simulink model "Mastership"  (R2013b)
settings: Solver=ode45  StartTime=0.0  StopTime=6e-4  RelTol=1e-3
(part 2 of 3)

== stateflow chart Mastership/MVBC/MVB3 ==
  state ClockManager [parallel]
    settings: executionOrder=1
    note: 描述：时钟管理模块，负责从主时钟（24Mhz）分频产生不同的时钟信号。同时负责过程数据
        | 更新时间戳的生成。
        | 通信方法：0.时钟频率24MHz, RST信号异步复位
        | 			1.3Mhz时钟输出：CLK_3Mhz
        | 			2.1Khz时钟输出：CLK_1Khz
        | 			3.时间戳输出：timeStamp（每1ms计数1次）
        | 假定情况：未考虑时钟同步提取问题，后期工作应加入设备间时钟同步模块
        | 作者：周彦钊
        | 最后修改者：周彦钊
        | 更新日期：2014.1.21
    state FreqDivider [parallel]
      settings: executionOrder=1
      note: 描述：分频器
      state Wait
        ClockManager.FreqDivider.Wait -> ClockManager.FreqDivider.Wait [order 1] : [!RST]
            | {Reset();}
      state Event
        (default) -> (junction 30)
        (junction 30) -> (junction 24) [order 1] : [counter_3M==4]
            | {CLK_3MHz=~CLK_3MHz
            | counter_3M=0;}
        (junction 30) -> (junction 33) [order 2]
        (junction 24) -> (junction 33)
        (junction 33) -> (junction 37) [order 1] : [counter_1K==12000]
            | {CLK_1KHz=~CLK_1KHz;
            | counter_1K=0;}
        (junction 33) -> (junction 386) [order 2]
        (junction 37) -> (junction 386)
        (junction 386) -> (junction 388) : [counter_BasicPeriod==100]
            | {basicPeriodStart = ~basicPeriodStart
            | counter_BasicPeriod = 0;}
      (default) -> ClockManager.FreqDivider.Wait : {Reset();}
      ClockManager.FreqDivider.Event -> ClockManager.FreqDivider.Wait
      ClockManager.FreqDivider.Wait -> ClockManager.FreqDivider.Event [order 1] : [hasChangedTo(CLK_24MHz, 1)]
          | {counter_3M++;
          | counter_1K++;
          | counter_BasicPeriod++;}
    state TimeStampGenerator [parallel]
      settings: executionOrder=2
      note: 描述：时间戳生成
      state Wait
        ClockManager.TimeStampGenerator.Wait -> ClockManager.TimeStampGenerator.Wait [order 1] : [!RST]{Reset();}
      state Event
        (junction 50) -> (junction 53) [order 1] : [timeStamp<4294967294]
            | {timeStamp++;}
        (junction 50) -> (junction 53) [order 2] : {Reset();}
        (default) -> (junction 50)
      (default) -> ClockManager.TimeStampGenerator.Wait : {Reset();}
      ClockManager.TimeStampGenerator.Event -> ClockManager.TimeStampGenerator.Wait
      ClockManager.TimeStampGenerator.Wait -> ClockManager.TimeStampGenerator.Event [order 1] : [hasChangedTo(CLK_1KHz,1)]
  state Sender [parallel]
    settings: executionOrder=2
    note: 描述：数据发送单元，具有CRC生成，Manchester编码，帧结构装配的功能
        | 通信方法：0.时钟频率3MHz
        | 			1.设置帧标志sendFrameTag：0为从帧，1为主帧
        | 			2.装入数据缓冲区sendDataBuf：uint16
        | 			3.使能发送sendEnable：低有效，数据从dataOut口串行发出，
        | 			   信息速率Rb为3Mbps
        | 			4.发送完成后根据发送类型，不同标志位将被置位，如：
        | 			    sendMasterFrame（主帧被发送，高有效）
        | 			    slaveMasterFrame（从帧被发送，高有效）
        | 假定情况：假设从帧发送数据最大长度为16bit，后续工作应支持16,32,64,128,256bit
        | 作者：周彦钊
        | 最后修改者：周彦钊
        | 更新日期：2014.1.21
    state FrameStructureControl [parallel]
      settings: executionOrder=1
      note: 描述：帧结构装配控制
      state Wait
        Sender.FrameStructureControl.Wait -> Sender.FrameStructureControl.Wait [order 1] : [!RST]{Reset();}
      state FrameHeader
        en:
        SetHeader();
        shiftEnable = 1;
      state FrameData
        en:
        SetData();
        shiftEnable = 1;
      state FrameTail
        en:
        SetTail();
        shiftEnable = 1;
      state Done
        ex:SetSendState();
      (default) -> Sender.FrameStructureControl.Wait : {Reset();}
      Done -> Sender.FrameStructureControl.Wait : [hasChangedTo(CLK_3MHz,1)]
      FrameTail -> Sender.FrameStructureControl.Wait [order 1] : [!RST]
      FrameData -> Sender.FrameStructureControl.Wait [order 1] : [!RST]
      FrameHeader -> Sender.FrameStructureControl.Wait [order 1] : [!RST]
      Sender.FrameStructureControl.Wait -> FrameHeader [order 1] : [!sendEnable]
      FrameHeader -> FrameData [order 2] : [!shiftEnable]
      FrameData -> FrameTail [order 2] : [!shiftEnable]
      FrameTail -> Done [order 2] : [!shiftEnable]
    state ShiftRegister [parallel]
      settings: executionOrder=2
      note: 描述：发送FIFO控制
      state Wait
        en:Reset();
      state Shift
        ex:shiftEnable=0;
        Shift -> Shift [order 1] : [hasChangedTo(CLK_3MHz,1) ]
            | {ShiftFIFO();counter++;}
      (default) -> Sender.ShiftRegister.Wait
      Shift -> Sender.ShiftRegister.Wait [order 1] : [counter==shiftCount]
      Sender.ShiftRegister.Wait -> Shift : [shiftEnable]{counter=0;}
  state Receiver [parallel]
    settings: executionOrder=3
    note: 描述：数据接收单元，具有帧头检测，Manchester译码，CRC校验，去帧头帧尾的功能，
        | 具有AB两路数据输入来源，根据接收状态自动选择信任线与监视线，具备检测总线
        | 寂静、冲突（接收长度错或CRC错）和主从帧超时的能力。
        | 通信方法：0.时钟频率24MHz
        | 			1.当收到有效帧后会将数据存入缓冲区recvDataBuf并产生对应的接收通知，
        | 			如：recvMasterFrame（收到主帧，高有效）
        | 				 recvSlaveFrame（收到从帧，高有效）
        | 			2.从上一个接收事件后总线寂静1.4ms则产生一个通知：silentBus(高有效)
        | 			3.从上一个主帧接收后1.3ms没有接到主帧则产生一个通知：MainFrameTimeOut(高有效)
        | 			4.从收到主帧后42.7us内没有收到从帧则产生一个通知：SlaveFrameTimeOut(高有效)
        | 			5.当trustLineA标记为1时，当前信任线为LineA，监督线为LineB，反之同理
        | 假定情况：假设从帧接收最大数据长度为16bit，后续工作应支持16,32,64,128,256bit
        | 作者：周彦钊
        | 最后修改者：周彦钊
        | 更新日期：2014.1.22
    state LineA [parallel]
      du:recvError = recvLenError || recvCRCError;
      settings: executionOrder=1
      note: 描述：线路A接收
      state HeaderDectect
        en:
        Reset();
        sampleBufLen=144;
        Receiver.LineA.HeaderDectect -> Receiver.LineA.HeaderDectect [order 1] : [hasChangedTo(CLK_24MHz,1)]
            | {
            | PushData();
            | DetectFrameHeader();
            | }
      state FrameDecode
        en:
        sampleBufLen=416;
        counter=0;
        state LengthDetect
          Receiver.LineA.FrameDecode.LengthDetect -> Receiver.LineA.FrameDecode.LengthDetect [order 1] : [hasChangedTo(CLK_24MHz,1)]
              | {
              | PushData();
              | counter++;
              | DetectFrameEnd();
              | }
        state DataCheck
          en:
          CheckData();
        (default) -> Receiver.LineA.FrameDecode.LengthDetect
        Receiver.LineA.FrameDecode.LengthDetect -> Receiver.LineA.FrameDecode.DataCheck [order 1] : [recvFrameEnd && !recvLenError]
      (default) -> Receiver.LineA.HeaderDectect
      Receiver.LineA.FrameDecode.DataCheck -> Receiver.LineA.HeaderDectect : [!pause]
      Receiver.LineA.FrameDecode -> Receiver.LineA.HeaderDectect : [hasChangedTo(recvError, 1)...
          | || !RST]
      Receiver.LineA.HeaderDectect -> Receiver.LineA.FrameDecode [order 1] : [recvMasterFrameHeader...
          | || recvSlaveFrameHeader]
    state LineB [parallel]
      du:recvError = recvLenError || recvCRCError;
      settings: executionOrder=2
      note: 描述：线路B接收
      state HeaderDectect
        en:
        Reset();
        sampleBufLen=144;
        Receiver.LineB.HeaderDectect -> Receiver.LineB.HeaderDectect [order 1] : [hasChangedTo(CLK_24MHz,1)]
            | {
            | PushData();
            | DetectFrameHeader();
            | }
      state FrameDecode
        en:
        sampleBufLen=416;
        counter=0;
        state LengthDetect
          Receiver.LineB.FrameDecode.LengthDetect -> Receiver.LineB.FrameDecode.LengthDetect [order 1] : [hasChangedTo(CLK_24MHz,1)]
              | {
              | PushData();
              | counter++;
              | DetectFrameEnd();
              | }
        state DataCheck
          en:
          CheckData();
        (default) -> Receiver.LineB.FrameDecode.LengthDetect
        Receiver.LineB.FrameDecode.LengthDetect -> Receiver.LineB.FrameDecode.DataCheck [order 1] : [recvFrameEnd && !recvLenError]
      (default) -> Receiver.LineB.HeaderDectect
      Receiver.LineB.FrameDecode.DataCheck -> Receiver.LineB.HeaderDectect : [!pause]
      Receiver.LineB.FrameDecode -> Receiver.LineB.HeaderDectect : [hasChangedTo(recvError, 1)...
          | || !RST]
      Receiver.LineB.HeaderDectect -> Receiver.LineB.FrameDecode [order 1] : [recvMasterFrameHeader...
          | || recvSlaveFrameHeader]
    state RecvController [parallel]
      settings: executionOrder=3
      note: 描述：接收控制器，根据AB线状态自动选择信任线与观察线，并负责监测总线寂静和主从帧超时
      state ABController [parallel]
        settings: executionOrder=1
        state Wait
          Receiver.RecvController.ABController.Wait -> Receiver.RecvController.ABController.Wait : [hasChangedTo(CLK_24MHz,1)]
              | {recvFrame=LineA.recvMasterFrame || LineA.recvSlaveFrame...
              | 				|| LineB.recvMasterFrame || LineB.recvSlaveFrame;
              | 	recvMFA = LineA.recvMasterFrame;
              | 	recvSFA = LineA.recvSlaveFrame;
              | 	recvMFB = LineB.recvMasterFrame;
              | 	recvSFB = LineB.recvSlaveFrame;
              | 	DataBufA = LineA.recvDataBuf;
              | 	DataBufB = LineB.recvDataBuf;
              |  	lineAError = LineA.recvLenError || LineA.recvCRCError;
              | 	lineBError = LineB.recvLenError || LineB.recvCRCError;
              | CheckLine();
              | LineA.pause=0;
              | LineB.pause=0;}
        (default) -> Receiver.RecvController.ABController.Wait : {trustLineA=1;recvMasterFrame=0;recvSlaveFrame=0;}
      state SilenceAndTimeoutDetect [parallel]
        settings: executionOrder=2
        state Wait
          ex:
          Step();
        state Event
          (default) -> (junction 228)
          (junction 228) -> (junction 192) [order 1] : [silenceCounter==4200]
              | {silentBus=1;}
          (junction 228) -> (junction 226) [order 2]
          (junction 192) -> (junction 226)
          (junction 226) -> (junction 232) [order 1] : [MFTimeoutCounter==75]
              | {masterFrameTimeout=1;}
          (junction 226) -> (junction 236) [order 2]
          (junction 232) -> (junction 236)
          (junction 236) -> (junction 239) : [SFTimeoutCounter==75]
              | {slaveFrameTimeout=1;}
        (default) -> Receiver.RecvController.SilenceAndTimeoutDetect.Wait : {Reset();}
        Receiver.RecvController.SilenceAndTimeoutDetect.Event -> Receiver.RecvController.SilenceAndTimeoutDetect.Wait [order 2]
        Receiver.RecvController.SilenceAndTimeoutDetect.Event -> Receiver.RecvController.SilenceAndTimeoutDetect.Wait [order 1] : [!RST]{Reset();}
        Receiver.RecvController.SilenceAndTimeoutDetect.Wait -> Receiver.RecvController.SilenceAndTimeoutDetect.Event : [hasChangedTo(CLK_3MHz,1)]
  state MainProc [parallel]
    settings: executionOrder=4
    note: 描述：主权转移功能模块，包含检测到总线寂静时的主权竞争（含主权冲突的处理）；正常的主权转移过程，
        | 主权转移被拒绝的处理过程
        | 执行过程：1.从模块等待，主模块从主帧池中取出主帧发送，等待从帧应答，根据不同的应答结果控制状态变化
        | 			2.检测到总线寂静时，根据BAList的索引值进行主权竞争
        | 假定情况：1.简化了与TM（通信存储器）的访问流程，以提高仿真速度，后期工作应使用握手协议通信
        | 			2.为了便于仿真演示，只包含宏周期的最后一个基本周期，即主权转移周期
        | 作者：周彦钊
        | 最后修改者：周彦钊
        | 更新日期：2014.1.22
    state Proc [parallel]
      settings: executionOrder=2
      state Wait
      state CheckMainFrame
        en:
        masterFrameASK=1;
      state SendMainFrame
        en:
        sendFrameTag = 1;
        sendDataBuf=mfDataBuf;
        sendEnable=0;
      state WaitMasterFrame
      state MasterFrameProc
        en:
        recvMasterFrame=0;
        MFProc();
      state StandUp
        state Wait
          MainProc.Proc.StandUp.Wait -> MainProc.Proc.StandUp.Wait [order 1] : [hasChangedTo(CLK_3MHz,1)]{counter--;}
        state BeMaster
          en:
          isMaster = 1;
        (default) -> MainProc.Proc.StandUp.Wait : {counter=(deviceID+1) * 105;}
        MainProc.Proc.StandUp.Wait -> BeMaster [order 1] : [counter==0]
      state WaitSlaveFrame
      state SlaveFrameProc
        en:
        recvSlaveFrame=0;
        SFProc();
      (default) -> MainProc.Proc.Wait
      SlaveFrameProc -> MainProc.Proc.Wait
      BeMaster -> MainProc.Proc.Wait
      WaitSlaveFrame -> MainProc.Proc.Wait [order 2] : [slaveFrameTimeout==1]{slaveFrameTimeout=0;}
      MainProc.Proc.Wait -> CheckMainFrame
      CheckMainFrame -> (junction 365) : [masterFrameASK==0]
      (junction 365) -> WaitMasterFrame [order 2]
      (junction 365) -> SendMainFrame [order 1] : [!mfPoolEmpty]
      SendMainFrame -> WaitMasterFrame
      WaitMasterFrame -> StandUp [order 2] : [masterFrameTimeout==1]{masterFrameTimeout=0;}
      WaitMasterFrame -> MasterFrameProc [order 1] : [recvMasterFrame==1]
      StandUp -> MasterFrameProc : [recvMasterFrame==1]
      MasterFrameProc -> WaitSlaveFrame
      WaitSlaveFrame -> SlaveFrameProc [order 1] : [recvSlaveFrame==1]
    state MasterFramePoolController [parallel]
      settings: executionOrder=1
      note: 描述：主帧池控制器，根据当前的状态确认主帧池内容，控制主从设备
          | 执行对应的功能
      state Wait
      state Event
        (default) -> (junction 348)
        (junction 348) -> (junction 351) [order 2] : {mfPoolEmpty=1;
            | masterFrameASK=0;}
        (junction 348) -> (junction 349) [order 1] : [isMaster]
            | {GetMasterFrame();
            | mfPoolEmpty=0;
            | masterFrameASK=0;}
      (default) -> MainProc.MasterFramePoolController.Wait : {Reset();}
      MainProc.MasterFramePoolController.Event -> MainProc.MasterFramePoolController.Wait [order 1] : [!RST]{Reset();}
      MainProc.MasterFramePoolController.Event -> MainProc.MasterFramePoolController.Wait [order 2]
      MainProc.MasterFramePoolController.Wait -> MainProc.MasterFramePoolController.Event : [hasChangedTo(masterFrameASK,1)]
  data: counter_3M local uint8 =0; counter_1K local uint32 =0; counter_BasicPeriod local uint16; counter local double; sendFIFO local uint32; shiftEnable local boolean; shiftCount local uint8; counter local uint16 =0; sampleBuf local boolean size=416; sampleBufLen local uint16; recvError local boolean; recvMasterFrameHeader local boolean; recvSlaveFrameHeader local boolean; recvFrameEnd local boolean; recvLenError local boolean; recvCRCError local boolean; recvDataBuf local uint16; recvMasterFrame local boolean; recvSlaveFrame local boolean; pause local boolean; counter local uint16 =0; sampleBuf local boolean size=416; sampleBufLen local uint16; recvError local boolean; recvMasterFrameHeader local boolean; recvSlaveFrameHeader local boolean; recvFrameEnd local boolean; recvLenError local boolean; recvCRCError local boolean; recvDataBuf local uint16; recvMasterFrame local boolean; recvSlaveFrame local boolean; pause local boolean; recvFrame local boolean; lineAError local boolean; lineBError local boolean; recvMFA local boolean; recvSFA local boolean; recvMFB local boolean; recvSFB local boolean; DataBufA local uint16; DataBufB local uint16; silenceCounter local uint32; MFTimeoutCounter local uint32; SFTimeoutCounter local uint32; SFCounterEnable local boolean; counter local uint32; baIndex local uint16; CLK_24MHz input boolean; RST input boolean; CLK_3MHz output boolean =false; CLK_1KHz output boolean =false; timeStamp local uint32 =0; sendFrameTag local boolean; sendDataBuf local uint16; sendEnable local boolean; dataOut output boolean =false; sendMasterFrame local boolean =false; sendSlaveFrame local boolean =false; dataInA input boolean; dataInB input boolean; silentBus local boolean =false; trustLineA local boolean =true; recvMasterFrame local boolean; recvSlaveFrame local boolean; recvDataBuf local uint16; masterFrameTimeout local boolean =false; slaveFrameTimeout local boolean =false; isMaster output boolean =false; masterFrameASK local boolean; mfPoolEmpty local boolean; masterFrameACK local boolean; deviceConfig input uint16; deviceState input uint16; transState output uint16 =0; basicPeriodStart local boolean; mfDataBuf local uint16; deviceID input uint16; maxDeviceCount parameter uint16
  function Reset:
    | function Reset
    |     counter_3M = uint8(0);
    |     counter_1K = uint32(0);
    |     counter_BasicPeriod = uint16(0);
    |     CLK_3MHz = true;
    |     CLK_1KHz = true;
    |     basicPeriodStart =false;
    | end
  function Reset:
    | function Reset
    |     timeStamp = uint32(0);
    | end
  function Reset:
    | function Reset
    |     shiftEnable = false;
    |     sendMasterFrame = false;
    |     sendSlaveFrame = false;
    |     sendEnable = true;
    | end
  function SetHeader:
    | function SetHeader
    |     if sendFrameTag
    |         sendFIFO = uint32(2982494208);
    |     else
    |         sendFIFO = uint32(2855845888);
    |     end
    |     shiftCount = uint8(18);
    | end
  function SetData:
    | function SetData
    |     sendFIFO = uint32(0);
    |     for i = 0:15
    |         step = uint32(1 + GetBit(sendDataBuf, 15 - i));
    |         sendFIFO = sendFIFO + uint32(bitshift(step, 2 * (15 - i)));
    |     end
    |     shiftCount = uint8(32);
    | end
    | 
    | function r = GetBit(num, index)
    |     r = bitand(bitshift(num,  - index), 1);
    | end
  function SetTail:
    | function SetTail
    |     sendFIFO = uint32(0);
    |     Tail = uint32(GetCheckCode);
    |     for i = 0:7
    |         step = uint32(1 + GetBit(Tail, 7 - i));
    |         sendFIFO = sendFIFO + uint32(bitshift(step, 2 * (7 - i)));
    |     end
    |     sendFIFO = bitshift(sendFIFO, 16);      %移到高位
    |     sendFIFO = bitor(sendFIFO, 12288);      %结束符0011
    |     shiftCount = uint8(20);                 %8位校验码编码后变成16位，再加0011结束符，共20位
    | end
    | 
    | function r = GetCheckCode
    |     tmp=zeros(1, 16);
    |     msg=dec2bin(sendDataBuf);
    |     [~, n] = size(msg);
    |     tmp((16-n+1):16) = msg - 48;
    |     msg = tmp;
    |     generator = [1 1 1 0 0 1 0 1];          % 7bit CRC生成多项式
    |     multip = conv([1 0 0 0 0 0 0 0 ], msg); % 左移7位
    |     [~, CRC] = deconv(multip, generator);   % 对多项式的除，就等于做反卷积 
    |     CRC = mod(CRC(end - 6: end), 2);        % 对除法的余数做模二运算
    |     CRC = CRC(end - 6: end);
    |     count = 0;
    |     for i = 1:length(CRC)
    |         if CRC(i)
    |             count = count + 1;
    |             CRC(i) = 0;
    |         else
    |             CRC(i) = 1;
    |         end
    |     end
    |     if mod(count, 2) == 0
    |         CRC = [CRC, 1];                  %添加0，但取反了
    |     else
    |         CRC = [CRC, 0];
    |     end
    |     r = uint32(GetDec(CRC));
    | end
    | 
    | function r = GetDec(b)
    |     r = 0;
    |     for i = 1: length(b)
    |         r = r + b(i) * power(2,(length(b) - i));
    |     end 
    | end
    | 
    | function r = GetBit(num, index)
    |     r = bitand(bitshift(num,  - index), 1);
    | end
  function SetSendState:
    | function SetSendState
    |     if sendFrameTag
    |         sendMasterFrame = true;
    |     else
    |         sendSlaveFrame = true;
    |     end
    |     sendEnable = true;
    |     dataOut = false;
    | end
  function ShiftFIFO:
    | function ShiftFIFO
    |     dataOut = GetHighBit;
    |     sendFIFO = bitshift(sendFIFO, 1);
    | end
    | 
    | function r = GetHighBit
    |    r = bitshift(sendFIFO, -31) == 1;
    | end
  function Reset:
    | function Reset
    |     sendFIFO = uint32(0);
    |     shiftCount = uint8(0);
    | end
  function DetectFrameHeader:
    | function DetectFrameHeader
    |     recvMasterFrameHeader = (checkEqual(sampleBuf(1:8),[1 1 1 1 1 1 1 1])...
    |            || checkEqual(sampleBuf(1:8),[1 1 1 1 1 1 1 0])...
    |            || checkEqual(sampleBuf(1:8),[1 1 1 1 1 1 0 1])...
    |            || checkEqual(sampleBuf(1:8),[1 1 1 1 1 0 1 1])...
    |            || checkEqual(sampleBuf(1:8),[1 1 1 1 0 1 1 1])...
    |            || checkEqual(sampleBuf(1:8),[1 1 1 0 1 1 1 1])...
    |            || checkEqual(sampleBuf(1:8),[1 1 0 1 1 1 1 1])...
    |            || checkEqual(sampleBuf(1:8),[1 0 1 1 1 1 1 1])...
    |            || checkEqual(sampleBuf(1:8),[0 1 1 1 1 1 1 1])...
    |            || checkEqual(sampleBuf(1:8),[0 0 1 1 1 1 1 1])...
    |            || checkEqual(sampleBuf(1:8),[1 1 1 1 1 1 0 0])...
    |            || checkEqual(sampleBuf(1:8),[0 1 1 1 1 1 1 0])...
    |            || checkEqual(sampleBuf(1:8),[0 0 1 1 1 1 0 0]))...
    |            && (checkEqual(sampleBuf(9:16),[0 0 0 0 0 0 0 1])...
    |            || checkEqual(sampleBuf(9:16),[0 0 0 0 0 0 1 0])...
    |            || checkEqual(sampleBuf(9:16),[0 0 0 0 0 1 0 0])...
    |            || checkEqual(sampleBuf(9:16),[0 0 0 0 1 0 0 0])...
    |            || checkEqual(sampleBuf(9:16),[0 0 0 1 0 0 0 0])...
    |            || checkEqual(sampleBuf(9:16),[0 0 1 0 0 0 0 0])...
    |            || checkEqual(sampleBuf(9:16),[0 1 0 0 0 0 0 0])...
    |            || checkEqual(sampleBuf(9:16),[1 0 0 0 0 0 0 0])...
    |            || checkEqual(sampleBuf(9:16),[1 1 0 0 0 0 0 0])...
    |            || checkEqual(sampleBuf(9:16),[0 0 0 0 0 0 1 1])...
    |            || checkEqual(sampleBuf(9:16),[1 0 0 0 0 0 0 1])...
    |            || checkEqual(sampleBuf(9:16),[1 1 0 0 0 0 1 1])...
    |            || checkEqual(sampleBuf(9:16),[0 0 0 0 0 0 0 0]))...
    |            && sampleBuf(21) && sampleBuf(29) && ~sampleBuf(37) && ~sampleBuf(45)...
    |            && ~sampleBuf(53) && sampleBuf(61) && sampleBuf(69) && sampleBuf(77)...
    |            && ~sampleBuf(85) && ~sampleBuf(93) && ~sampleBuf(101) && sampleBuf(109)...
    |            && ~sampleBuf(117) && sampleBuf(125) && ~sampleBuf(133) && sampleBuf(141);
    |       if ~recvMasterFrameHeader
    |           recvSlaveFrameHeader = (checkEqual(sampleBuf(1:8),[1 1 1 1 1 1 1 1])...
    |            || checkEqual(sampleBuf(1:8),[1 1 1 1 1 1 1 0])...
    |            || checkEqual(sampleBuf(1:8),[1 1 1 1 1 1 0 1])...
    |            || checkEqual(sampleBuf(1:8),[1 1 1 1 1 0 1 1])...
    |            || checkEqual(sampleBuf(1:8),[1 1 1 1 0 1 1 1])...
    |            || checkEqual(sampleBuf(1:8),[1 1 1 0 1 1 1 1])...
    |            || checkEqual(sampleBuf(1:8),[1 1 0 1 1 1 1 1])...
    |            || checkEqual(sampleBuf(1:8),[1 0 1 1 1 1 1 1])...
    |            || checkEqual(sampleBuf(1:8),[0 1 1 1 1 1 1 1])...
    |            || checkEqual(sampleBuf(1:8),[0 0 1 1 1 1 1 1])...
    |            || checkEqual(sampleBuf(1:8),[1 1 1 1 1 1 0 0])...
    |            || checkEqual(sampleBuf(1:8),[0 1 1 1 1 1 1 0])...
    |            || checkEqual(sampleBuf(1:8),[0 0 1 1 1 1 0 0]))...
    |            && (checkEqual(sampleBuf(9:16),[0 0 0 0 0 0 0 1])...
    |            || checkEqual(sampleBuf(9:16),[0 0 0 0 0 0 1 0])...
    |            || checkEqual(sampleBuf(9:16),[0 0 0 0 0 1 0 0])...
    |            || checkEqual(sampleBuf(9:16),[0 0 0 0 1 0 0 0])...
    |            || checkEqual(sampleBuf(9:16),[0 0 0 1 0 0 0 0])...
    |            || checkEqual(sampleBuf(9:16),[0 0 1 0 0 0 0 0])...
    |            || checkEqual(sampleBuf(9:16),[0 1 0 0 0 0 0 0])...
    |            || checkEqual(sampleBuf(9:16),[1 0 0 0 0 0 0 0])...
    |            || checkEqual(sampleBuf(9:16),[1 1 0 0 0 0 0 0])...
    |            || checkEqual(sampleBuf(9:16),[0 0 0 0 0 0 1 1])...
    |            || checkEqual(sampleBuf(9:16),[1 0 0 0 0 0 0 1])...
    |            || checkEqual(sampleBuf(9:16),[1 1 0 0 0 0 1 1])...
    |            || checkEqual(sampleBuf(9:16),[0 0 0 0 0 0 0 0]))...
    |            && sampleBuf(21) && ~sampleBuf(29) && sampleBuf(37) && ~sampleBuf(45)...
    |            && sampleBuf(53) && ~sampleBuf(61) && ~sampleBuf(69) && ~sampleBuf(77)...
    |            && sampleBuf(85) && sampleBuf(93) && sampleBuf(101) && ~sampleBuf(109)...
    |            && ~sampleBuf(117) && ~sampleBuf(125) && sampleBuf(133) && sampleBuf(141);
    |       end
    | end
    |  
    | function r = checkEqual(a, b)
    |     r = length(a)==length(b);
    |     if r
    |         for i = 1:length(a)
    |             if a(i) ~= b(i)
    |                 r = false;
    |                 break;
    |             end
    |         end
    |     end
    | end
  function Reset:
    | function Reset
    |     for i = 1:length(sampleBuf)
    |         sampleBuf(i) = false;
    |     end
    |     recvMasterFrameHeader = false;
    |     recvSlaveFrameHeader = false;
    |     recvFrameEnd = false;
    |     recvLenError = false;
    |     recvCRCError = false;
    |     recvMasterFrame = false;
    |     recvSlaveFrame = false;
    |     pause = false;
    | end
  function PushData:
    | function PushData
    |     for i = 1: sampleBufLen - 1
    |         sampleBuf(i) = sampleBuf(i + 1);
    |     end
    |     sampleBuf(sampleBufLen) = dataInA;
    | end
  function CheckData:
    | function CheckData
    |     recvCRCError = false;
    |     tmp = zeros(1, 48);
    |     %采样判决
    |     for i = 1: length(tmp)
    |         tmp(i) = uint8(sampleBuf(5 + 8 * (i - 1)));
    |     end
    |     
    |     code = zeros(1, 24);
    |     %Manchester译码
    |     for i = 1: length(code)
    |         j = 2 * ( i - 1) + 1;
    |         if (tmp(j) == 0) && (tmp(j + 1) == 1)
    |             code(i) = uint8(0);
    |         elseif (tmp(j) == 1) && (tmp(j + 1) == 0)
    |             code(i) = uint8(1);
    |         else
    |             recvCRCError = true;   %非0 1字符
    |         end
    |     end
    |     
    |     %偶校验
    |     evenBitCount = 0;
    |     for i = 17: 24
    |         if code(i)
    |             code(i) = 0;
    |         else
    |             code(i) = 1;
    |             evenBitCount = evenBitCount + 1;
    |         end
    |     end
    |     
    |     if mod(evenBitCount, 2) == 0
    |         %CRC校验
    |         generator = [1 1 1 0 0 1 0 1];
    |         [~, remainder]=deconv(code(1: end - 1), generator);	
    |         remainder=mod(remainder(end - 6: end), 2);
    |         if isequal(remainder,[0 0 0 0 0 0 0])
    |             recvDataBuf = uint16(GetDec(code(1: 16)));
    |             recvMasterFrame = recvMasterFrameHeader;
    |             recvSlaveFrame = recvSlaveFrameHeader;
    |         else
    |             recvCRCError = true;
    |         end
    |     else
    |         recvCRCError = true;
    |     end    
    |     pause = true; %暂停，等待控制器判决
    | end
    | 
    | function r = GetDec(b)
    |     r = 0;
    |     for i = 1: length(b)
    |         r = r + b(i) * power(2,(length(b) - i));
    |     end 
    | end
  function DetectFrameEnd:
    | function DetectFrameEnd
    |     if counter >= 416
    | %       结束符NL,NH检测
    |         recvFrameEnd = (checkEqual(sampleBuf(385:400),[0 0 0 0 0 0 0 0 0 0 0 0 0 0 0 0])...
    |            || checkEqual(sampleBuf(385:400),[1 1 0 0 0 0 0 0 0 0 0 0 0 0 1 1])...
    |            || checkEqual(sampleBuf(385:400),[1 0 0 0 0 0 0 0 0 0 0 0 0 0 0 1])...
    |            || checkEqual(sampleBuf(385:400),[1 0 0 0 0 0 0 0 0 0 0 0 0 0 1 1])...
    |            || checkEqual(sampleBuf(385:400),[1 1 0 0 0 0 0 0 0 0 0 0 0 0 0 1]))...
    |            && (checkEqual(sampleBuf(401:416),[1 1 1 1 1 1 1 1 1 1 1 1 1 1 1 1])...
    |            || checkEqual(sampleBuf(401:416),[0 0 1 1 1 1 1 1 1 1 1 1 1 1 0 0])...
    |            || checkEqual(sampleBuf(401:416),[0 1 1 1 1 1 1 1 1 1 1 1 1 1 1 0])...
    |            || checkEqual(sampleBuf(401:416),[0 1 1 1 1 1 1 1 1 1 1 1 1 1 0 0])...
    |            || checkEqual(sampleBuf(401:416),[0 0 1 1 1 1 1 1 1 1 1 1 1 1 1 0]));
    |          
    |             recvLenError = (counter > 416 + 4);        %允许延迟4个CLK为容错考虑
    |     end
    | end
    |  
    | function r = checkEqual(a, b)
    |     r = length(a)==length(b);
    |     if r
    |         for i = 1:length(a)
    |             if a(i) ~= b(i)
    |                 r = false;
    |                 break;
    |             end
    |         end
    |     end
    | end
  function DetectFrameHeader:
    | function DetectFrameHeader
    |     recvMasterFrameHeader = (checkEqual(sampleBuf(1:8),[1 1 1 1 1 1 1 1])...
    |            || checkEqual(sampleBuf(1:8),[1 1 1 1 1 1 1 0])...
    |            || checkEqual(sampleBuf(1:8),[1 1 1 1 1 1 0 1])...
    |            || checkEqual(sampleBuf(1:8),[1 1 1 1 1 0 1 1])...
    |            || checkEqual(sampleBuf(1:8),[1 1 1 1 0 1 1 1])...
    |            || checkEqual(sampleBuf(1:8),[1 1 1 0 1 1 1 1])...
    |            || checkEqual(sampleBuf(1:8),[1 1 0 1 1 1 1 1])...
    |            || checkEqual(sampleBuf(1:8),[1 0 1 1 1 1 1 1])...
    |            || checkEqual(sampleBuf(1:8),[0 1 1 1 1 1 1 1])...
    |            || checkEqual(sampleBuf(1:8),[0 0 1 1 1 1 1 1])...
    |            || checkEqual(sampleBuf(1:8),[1 1 1 1 1 1 0 0])...
    |            || checkEqual(sampleBuf(1:8),[0 1 1 1 1 1 1 0])...
    |            || checkEqual(sampleBuf(1:8),[0 0 1 1 1 1 0 0]))...
    |            && (checkEqual(sampleBuf(9:16),[0 0 0 0 0 0 0 1])...
    |            || checkEqual(sampleBuf(9:16),[0 0 0 0 0 0 1 0])...
    |            || checkEqual(sampleBuf(9:16),[0 0 0 0 0 1 0 0])...
    |            || checkEqual(sampleBuf(9:16),[0 0 0 0 1 0 0 0])...
    |            || checkEqual(sampleBuf(9:16),[0 0 0 1 0 0 0 0])...
    |            || checkEqual(sampleBuf(9:16),[0 0 1 0 0 0 0 0])...
    |            || checkEqual(sampleBuf(9:16),[0 1 0 0 0 0 0 0])...
    |            || checkEqual(sampleBuf(9:16),[1 0 0 0 0 0 0 0])...
    |            || checkEqual(sampleBuf(9:16),[1 1 0 0 0 0 0 0])...
    |            || checkEqual(sampleBuf(9:16),[0 0 0 0 0 0 1 1])...
    |            || checkEqual(sampleBuf(9:16),[1 0 0 0 0 0 0 1])...
    |            || checkEqual(sampleBuf(9:16),[1 1 0 0 0 0 1 1])...
    |            || checkEqual(sampleBuf(9:16),[0 0 0 0 0 0 0 0]))...
    |            && sampleBuf(21) && sampleBuf(29) && ~sampleBuf(37) && ~sampleBuf(45)...
    |            && ~sampleBuf(53) && sampleBuf(61) && sampleBuf(69) && sampleBuf(77)...
    |            && ~sampleBuf(85) && ~sampleBuf(93) && ~sampleBuf(101) && sampleBuf(109)...
    |            && ~sampleBuf(117) && sampleBuf(125) && ~sampleBuf(133) && sampleBuf(141);
    |       if ~recvMasterFrameHeader
    |           recvSlaveFrameHeader = (checkEqual(sampleBuf(1:8),[1 1 1 1 1 1 1 1])...
    |            || checkEqual(sampleBuf(1:8),[1 1 1 1 1 1 1 0])...
    |            || checkEqual(sampleBuf(1:8),[1 1 1 1 1 1 0 1])...
    |            || checkEqual(sampleBuf(1:8),[1 1 1 1 1 0 1 1])...
    |            || checkEqual(sampleBuf(1:8),[1 1 1 1 0 1 1 1])...
    |            || checkEqual(sampleBuf(1:8),[1 1 1 0 1 1 1 1])...
    |            || checkEqual(sampleBuf(1:8),[1 1 0 1 1 1 1 1])...
    |            || checkEqual(sampleBuf(1:8),[1 0 1 1 1 1 1 1])...
    |            || checkEqual(sampleBuf(1:8),[0 1 1 1 1 1 1 1])...
    |            || checkEqual(sampleBuf(1:8),[0 0 1 1 1 1 1 1])...
    |            || checkEqual(sampleBuf(1:8),[1 1 1 1 1 1 0 0])...
    |            || checkEqual(sampleBuf(1:8),[0 1 1 1 1 1 1 0])...
    |            || checkEqual(sampleBuf(1:8),[0 0 1 1 1 1 0 0]))...
    |            && (checkEqual(sampleBuf(9:16),[0 0 0 0 0 0 0 1])...
    |            || checkEqual(sampleBuf(9:16),[0 0 0 0 0 0 1 0])...
    |            || checkEqual(sampleBuf(9:16),[0 0 0 0 0 1 0 0])...
    |            || checkEqual(sampleBuf(9:16),[0 0 0 0 1 0 0 0])...
    |            || checkEqual(sampleBuf(9:16),[0 0 0 1 0 0 0 0])...
    |            || checkEqual(sampleBuf(9:16),[0 0 1 0 0 0 0 0])...
    |            || checkEqual(sampleBuf(9:16),[0 1 0 0 0 0 0 0])...
    |            || checkEqual(sampleBuf(9:16),[1 0 0 0 0 0 0 0])...
    |            || checkEqual(sampleBuf(9:16),[1 1 0 0 0 0 0 0])...
    |            || checkEqual(sampleBuf(9:16),[0 0 0 0 0 0 1 1])...
    |            || checkEqual(sampleBuf(9:16),[1 0 0 0 0 0 0 1])...
    |            || checkEqual(sampleBuf(9:16),[1 1 0 0 0 0 1 1])...
    |            || checkEqual(sampleBuf(9:16),[0 0 0 0 0 0 0 0]))...
    |            && sampleBuf(21) && ~sampleBuf(29) && sampleBuf(37) && ~sampleBuf(45)...
    |            && sampleBuf(53) && ~sampleBuf(61) && ~sampleBuf(69) && ~sampleBuf(77)...
    |            && sampleBuf(85) && sampleBuf(93) && sampleBuf(101) && ~sampleBuf(109)...
    |            && ~sampleBuf(117) && ~sampleBuf(125) && sampleBuf(133) && sampleBuf(141);
    |       end
    | end
    |  
    | function r = checkEqual(a, b)
    |     r = length(a)==length(b);
    |     if r
    |         for i = 1:length(a)
    |             if a(i) ~= b(i)
    |                 r = false;
    |                 break;
    |             end
    |         end
    |     end
    | end
  function Reset:
    | function Reset
    |     for i = 1:length(sampleBuf)
    |         sampleBuf(i) = false;
    |     end
    |     recvMasterFrameHeader = false;
    |     recvSlaveFrameHeader = false;
    |     recvFrameEnd = false;
    |     recvLenError = false;
    |     recvCRCError = false;
    |     recvMasterFrame = false;
    |     recvSlaveFrame = false;
    |     pause = false;
    | end
  function PushData:
    | function PushData
    |     for i = 1: sampleBufLen - 1
    |         sampleBuf(i) = sampleBuf(i + 1);
    |     end
    |     sampleBuf(sampleBufLen) = dataInB;
    | end
  function CheckData:
    | function CheckData
    |     recvCRCError = false;
    |     tmp = zeros(1, 48);
    |     %采样判决
    |     for i = 1: length(tmp)
    |         tmp(i) = uint8(sampleBuf(5 + 8 * (i - 1)));
    |     end
    |     
    |     code = zeros(1, 24);
    |     %Manchester译码
    |     for i = 1: length(code)
    |         j = 2 * ( i - 1) + 1;
    |         if (tmp(j) == 0) && (tmp(j + 1) == 1)
    |             code(i) = uint8(0);
    |         elseif (tmp(j) == 1) && (tmp(j + 1) == 0)
    |             code(i) = uint8(1);
    |         else
    |             recvCRCError = true;   %非0 1字符
    |         end
    |     end
    |     
    |     %偶校验
    |     evenBitCount = 0;
    |     for i = 17: 24
    |         if code(i)
    |             code(i) = 0;
    |         else
    |             code(i) = 1;
    |             evenBitCount = evenBitCount + 1;
    |         end
    |     end
    |     
    |     if mod(evenBitCount, 2) == 0
    |         %CRC校验
    |         generator = [1 1 1 0 0 1 0 1];
    |         [~, remainder]=deconv(code(1: end - 1), generator);	
    |         remainder=mod(remainder(end - 6: end), 2);
    |         if isequal(remainder,[0 0 0 0 0 0 0])
    |             recvDataBuf = uint16(GetDec(code(1: 16)));
    |             recvMasterFrame = recvMasterFrameHeader;
    |             recvSlaveFrame = recvSlaveFrameHeader;
    |         else
    |             recvCRCError = true;
    |         end
    |     else
    |         recvCRCError = true;
    |     end    
    |     pause = true; %暂停，等待控制器判决
    | end
    | 
    | function r = GetDec(b)
    |     r = 0;
    |     for i = 1: length(b)
    |         r = r + b(i) * power(2,(length(b) - i));
    |     end 
    | end
  function DetectFrameEnd:
    | function DetectFrameEnd
    |     if counter >= 416
    | %       结束符NL,NH检测
    |         recvFrameEnd = (checkEqual(sampleBuf(385:400),[0 0 0 0 0 0 0 0 0 0 0 0 0 0 0 0])...
    |            || checkEqual(sampleBuf(385:400),[1 1 0 0 0 0 0 0 0 0 0 0 0 0 1 1])...
    |            || checkEqual(sampleBuf(385:400),[1 0 0 0 0 0 0 0 0 0 0 0 0 0 0 1])...
    |            || checkEqual(sampleBuf(385:400),[1 0 0 0 0 0 0 0 0 0 0 0 0 0 1 1])...
    |            || checkEqual(sampleBuf(385:400),[1 1 0 0 0 0 0 0 0 0 0 0 0 0 0 1]))...
    |            && (checkEqual(sampleBuf(401:416),[1 1 1 1 1 1 1 1 1 1 1 1 1 1 1 1])...
    |            || checkEqual(sampleBuf(401:416),[0 0 1 1 1 1 1 1 1 1 1 1 1 1 0 0])...
    |            || checkEqual(sampleBuf(401:416),[0 1 1 1 1 1 1 1 1 1 1 1 1 1 1 0])...
    |            || checkEqual(sampleBuf(401:416),[0 1 1 1 1 1 1 1 1 1 1 1 1 1 0 0])...
    |            || checkEqual(sampleBuf(401:416),[0 0 1 1 1 1 1 1 1 1 1 1 1 1 1 0]));
    |          
    |             recvLenError = (counter > 416 + 4);        %允许延迟4个CLK为容错考虑
    |     end
    | end
    |  
    | function r = checkEqual(a, b)
    |     r = length(a)==length(b);
    |     if r
    |         for i = 1:length(a)
    |             if a(i) ~= b(i)
    |                 r = false;
    |                 break;
    |             end
    |         end
    |     end
    | end
  function CheckLine:
    | function CheckLine
    |   %信任线校正
    |   if trustLineA 
    |       %信任线异常时切换
    |       if lineAError
    |           trustLineA = false;
    |       end
    |       %信任线未收到数据而观察线收到数据时切换
    |       if ~(recvMFA || recvSFA) && (recvMFB || recvSFB)
    |           trustLineA = false;
    |       end
    |   else
    |       if lineBError
    |           trustLineA = true;
    |       end
    |       if ~(recvMFB || recvSFB) && (recvMFA || recvSFA)
    |           trustLineA = true;
    |       end
    |   end
    |   %总线寂静时切换
    |   if silentBus 
    |       trustLineA = ~trustLineA;
    |   end
    |   %读取信任线状态
    |   if trustLineA 
    |       %从A线读取
    |       if recvMFA
    |           recvDataBuf = DataBufA;
    |           silenceCounter = uint32(0);
    |           MFTimeoutCounter = uint32(0);
    |           SFTimeoutCounter = uint32(0);
    |           SFCounterEnable = true;
    |           recvMasterFrame = true;
    |       elseif recvSFA
    |           recvDataBuf = DataBufA;
    |           SFTimeoutCounter = uint32(0);
    |           SFCounterEnable = false;
    |           recvSlaveFrame = true;
    |       end
    |   else
    |       %从B线读取
    |       recvDataBuf = DataBufB;
    |       if recvMFB
    |           recvDataBuf = DataBufB;
    |           silenceCounter = uint32(0);
    |            MFTimeoutCounter = uint32(0);
    |            SFTimeoutCounter = uint32(0);
    |            SFCounterEnable = true;
    |           recvMasterFrame = true;
    |       elseif recvSFB
    |           recvDataBuf = DataBufB;
    |           SFTimeoutCounter = uint32(0);
    |           SFCounterEnable = false;
    |           recvSlaveFrame = true;
    |       end
    |   end
    | end
  function Reset:
    | function Reset
    |  SFTimeoutCounter = uint32(0);
    |  MFTimeoutCounter = uint32(0);
    |  silenceCounter = uint32(0);
    |  SFCounterEnable = false;
    | end
  function Step:
    | function Step
    |  MFTimeoutCounter = MFTimeoutCounter + 1;
    |  silenceCounter = silenceCounter + 1;
    |  if SFCounterEnable
    |      SFTimeoutCounter = SFTimeoutCounter + 1;
    |  end
    | end
  function MFProc:
    | function MFProc
    |     if isMaster && ~sendMasterFrame   %收到非自己发送的主帧，产生主权冲突
    |         isMaster = false;
    |     else
    |         tmp = recvDataBuf;
    |         tag = bitshift(tmp, -12);
    |         tmp = bitand(tmp, 4095);
    |         if tmp == deviceID
    |             sendFrameTag = false;
    |             switch(tag)
    |                 case 15     %状态查询
    |                     sendDataBuf = deviceState +61440;
    |                     sendEnable = false;
    |                 case  8     %转移请求
    |                     sendDataBuf = deviceConfig + 32768;
    |                     sendEnable = false;
    |                     if deviceConfig == 1
    |                         isMaster = true;
    |                     else
    |                         isMaster = false;
    |                     end
    |             end
    |         end
    |     end
    | end
  function SFProc:
    | function SFProc
    |     if isMaster
    |         tmp = recvDataBuf;
    |         tag = bitshift(tmp, -12);
    |         tmp = bitand(tmp, 4095);
    |         switch(tag)
    |                 case 15     %状态查询
    |                    if tmp
    |                        transState = uint16(1);      %符合条件
    |                    end
    |                 case  8     %转移请求
    |                     if tmp && transState == uint16(1)
    |                         isMaster = false;    %转移成功，放弃主权
    |                     end
    |                     transState = uint16(0);             
    |             end
    |     end
    | end
  function Reset:
    | function Reset
    |  baIndex = deviceID;
    | end
  function GetMasterFrame:
    | function GetMasterFrame
    | switch(transState)
    |     case 0  %条件查询
    |         baIndex = uint16(mod(baIndex + 1, maxDeviceCount));
    |         if baIndex == deviceID
    |             baIndex = uint16(mod(baIndex + 1, maxDeviceCount));
    |         end
    |         mfDataBuf = baIndex + uint16(61440);
    |     case 1  %条件符合时，主权移交
    |         mfDataBuf = baIndex + uint16(32768);
    |      end
    | end
